simulink model "TryControl1"  (R2021a)
settings: Solver=VariableStepAuto  StartTime=0.0  StopTime=8.0  RelTol=1e-3
undefined symbols (not defined in the file or in its folder): square
libraries: simulink x1
settings Model: Creator=Ziad Elbouriny  LastModifiedBy=Ziad Elbouriny

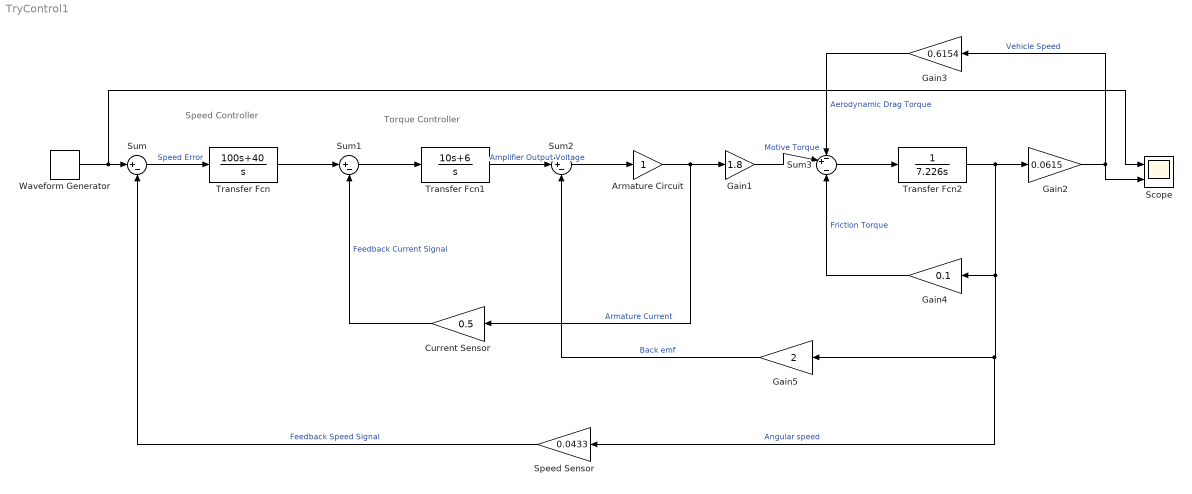
== system TryControl1 ==
  note: Torque Controller
  note: Speed Controller
  Armature Circuit : Gain
  Current Sensor : Gain  Gain=0.5
  Gain1 : Gain  Gain=1.8
  Gain2 : Gain  Gain=0.0615
  Gain3 : Gain  Gain=0.6154
  Gain4 : Gain  Gain=0.1
  Gain5 : Gain  Gain=2
  Scope : Scope  NumInputPorts=2
  Speed Sensor : Gain  Gain=0.0433
  Sum : Sum  Inputs=|+-
  Sum1 : Sum  Inputs=|+-
  Sum2 : Sum  Inputs=|+-
  Sum3 : Sum  Inputs=-+|-
  Transfer Fcn : TransferFcn  Numerator=[100 40]  Denominator=[1 0]
  Transfer Fcn1 : TransferFcn  Numerator=[10 6]  Denominator=[1 0]
  Transfer Fcn2 : TransferFcn  Denominator=[7.226 0]
  Waveform Generator : simulink/Sources/Waveform Generator  OutMin=[]  OutMax=[]  OutDataTypeStr=double  SelectedSignal=1  Signals=square('Amplitude',1,'Frequency',62,'Phase',0,'DutyCycle',50)  BlockNames=MultiportSwitch_b7967aa1dc6b469  SampleTime=0.001
  wires:
  Sum/1 -> Transfer Fcn/1  "Speed Error"
  Sum1/1 -> Transfer Fcn1/1
  Transfer Fcn/1 -> Sum1/1
  Transfer Fcn1/1 -> Sum2/1  "Amplifier Output Voltage"
  Sum2/1 -> Armature Circuit/1
  Armature Circuit/1 -> Current Sensor/1, Gain1/1  "Armature Current"
  Gain1/1 -> Sum3/2  "Motive Torque"
  Sum3/1 -> Transfer Fcn2/1
  Transfer Fcn2/1 -> Speed Sensor/1, Gain5/1, Gain4/1, Gain2/1  "Angular speed"
  Gain2/1 -> Gain3/1, Scope/2  "Vehicle Speed"
  Gain3/1 -> Sum3/1  "Aerodynamic Drag Torque"
  Gain4/1 -> Sum3/3  "Friction Torque"
  Gain5/1 -> Sum2/2  "Back emf"
  Speed Sensor/1 -> Sum/2  "Feedback Speed Signal"
  Current Sensor/1 -> Sum1/2  "Feedback Current Signal"
  Waveform Generator/1 -> Sum/1, Scope/1
